simulink model "program_flight"  (R2017a)
settings: Solver=ode4  StartTime=0.0  StopTime=10  FixedStep=0.001  RelTol=1e-3
InitFcn:
  | BeforeSim
values from neighbouring files (symbols this model uses):
  S_ref = pi*(0.5*d_ref)^2    (= 0.0702153812059)    [BeforeSim.m]
libraries: simulink_need_slupdate x12, simulink x1
settings Model: Creator=Hans  LastModifiedBy=hhz
settings OptimizationCC: LifeSpan=inf
settings DebuggingCC: SFExecutionAtInitializationDiag=none
settings HardwareCC: ProdBitPerSizeT=32  ProdBitPerPtrDiffT=32  ProdWordSize=32  ProdHWDeviceType=Specified

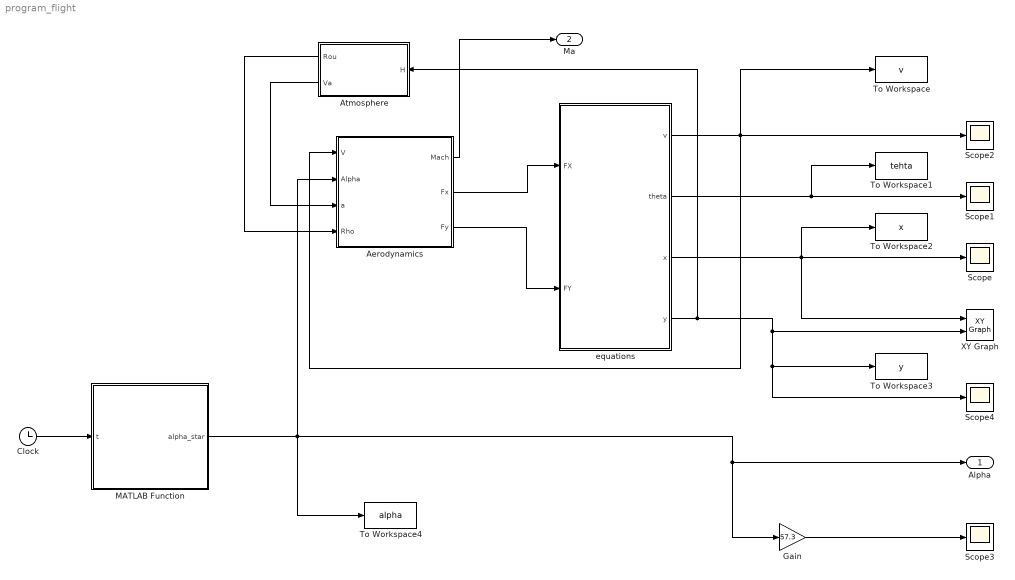
== system program_flight ==
  Aerodynamics : Subsystem
  Atmosphere : Subsystem
  Clock : Clock
  Gain : Gain  Gain=57.3
  MATLAB Function : MATLAB Function  TreatAsAtomicUnit=on
  Scope{,1..4} (5 alike) : Scope
  To Workspace : ToWorkspace  VariableName=v  SaveFormat=Timeseries  SampleTime=-1
  To Workspace1 : ToWorkspace  VariableName=tehta  SaveFormat=Timeseries  SampleTime=-1
  To Workspace2 : ToWorkspace  VariableName=x  SaveFormat=Timeseries  SampleTime=-1
  To Workspace3 : ToWorkspace  VariableName=y  SaveFormat=Timeseries  SampleTime=-1
  To Workspace4 : ToWorkspace  VariableName=alpha  SaveFormat=Timeseries  SampleTime=-1
  XY Graph : simulink/Sinks/XY Graph  xmin=0  xmax=3000  ymin=3000  ymax=4500  st=-1
  equations : Subsystem
  Alpha : Outport
  Ma : Outport  Port=2
  wires:
  Gain/1 -> Scope3/1
  equations/4(y) -> To Workspace3/1, Scope4/1, XY Graph/2, Atmosphere/1(H)
  equations/1(v) -> To Workspace/1, Scope2/1, Aerodynamics/1(V)
  Aerodynamics/1(" Mach") -> Ma/1
  Aerodynamics/2(Fx) -> equations/1(FX)
  Atmosphere/1(Rou) -> Aerodynamics/4(Rho)
  Aerodynamics/3(Fy) -> equations/2(FY)
  Atmosphere/2(Va) -> Aerodynamics/3(a)
  Clock/1 -> MATLAB Function/1(t)
  equations/2(theta) -> To Workspace1/1, Scope1/1
  equations/3(x) -> To Workspace2/1, XY Graph/1, Scope/1
  MATLAB Function/1(alpha_star) -> To Workspace4/1, Aerodynamics/2(Alpha), Alpha/1, Gain/1

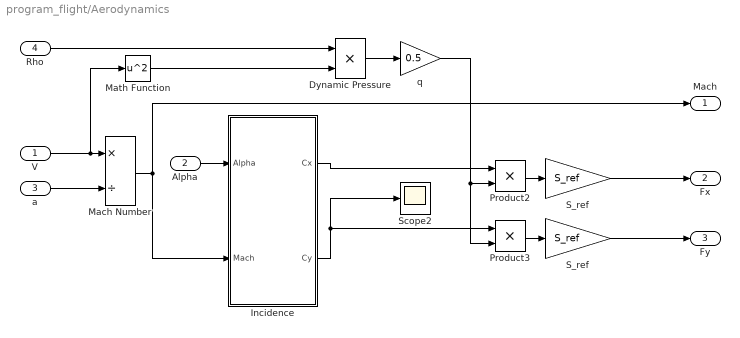
== system program_flight/Aerodynamics ==
  V : Inport
  Alpha : Inport  Port=2
  a : Inport  Port=3
  Rho : Inport  Port=4
  Dynamic Pressure : Product  SaturateOnIntegerOverflow=on  InputSameDT=on  OutDataTypeStr=Inherit: Same as first input
  Incidence : Subsystem
  Mach Number : Product  Inputs=*/  SaturateOnIntegerOverflow=on  InputSameDT=on  OutDataTypeStr=Inherit: Same as first input
  Math Function : Math  Operator=square  SaturateOnIntegerOverflow=on
  Product2 : Product  SaturateOnIntegerOverflow=on  InputSameDT=on  OutDataTypeStr=Inherit: Same as first input
  Product3 : Product  SaturateOnIntegerOverflow=on  InputSameDT=on  OutDataTypeStr=Inherit: Same as first input
  S_ref : Gain  Gain=S_ref  SaturateOnIntegerOverflow=on  OutDataTypeStr=Inherit: Same as input  ParamDataTypeStr=Inherit: Same as input
  "S_ref " : Gain  Gain=S_ref  SaturateOnIntegerOverflow=on  OutDataTypeStr=Inherit: Same as input  ParamDataTypeStr=Inherit: Same as input
  Scope2 : Scope
  q : Gain  Gain=0.5  SaturateOnIntegerOverflow=on  OutDataTypeStr=Inherit: Same as input  ParamDataTypeStr=Inherit: Same as input
  " Mach" : Outport  InitialOutput=0
  Fx : Outport  Port=2  InitialOutput=[0]
  Fy : Outport  Port=3  InitialOutput=0
  wires:
  Incidence/2(Cy) -> Product3/1, Scope2/1
  Product3/1 -> "S_ref "/1
  S_ref/1 -> Fx/1
  "S_ref "/1 -> Fy/1
  V/1 -> Math Function/1, Mach Number/1
  Alpha/1 -> Incidence/1(Alpha)
  Product2/1 -> S_ref/1
  Mach Number/1 -> " Mach"/1, Incidence/2(Mach)
  a/1 -> Mach Number/2
  q/1 -> Product2/2, Product3/2
  Rho/1 -> Dynamic Pressure/1
  Dynamic Pressure/1 -> q/1
  Math Function/1 -> Dynamic Pressure/2
  Incidence/1(Cx) -> Product2/1

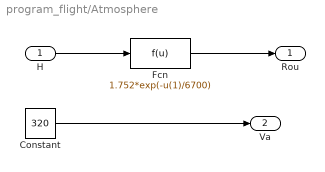
== system program_flight/Atmosphere ==
  H : Inport
  Constant : Constant  Value=320
  Fcn : Fcn  Expr=1.752*exp(-u(1)/6700)
  Rou : Outport
  Va : Outport  Port=2
  wires:
  H/1 -> Fcn/1
  Fcn/1 -> Rou/1
  Constant/1 -> Va/1

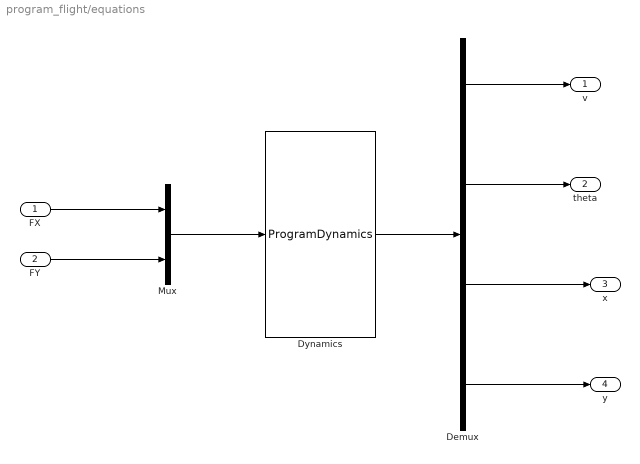
== system program_flight/equations ==
  FX : Inport
  FY : Inport  Port=2
  Demux : Demux
  Dynamics : S-Function  FunctionName=ProgramDynamics  SFunctionDeploymentMode=off  EnableBusSupport=off
  Mux : Mux  Inputs=2
  v : Outport
  theta : Outport  Port=2
  x : Outport  Port=3
  y : Outport  Port=4
  wires:
  FX/1 -> Mux/1
  FY/1 -> Mux/2
  Mux/1 -> Dynamics/1
  Dynamics/1 -> Demux/1
  Demux/1 -> v/1
  Demux/2 -> theta/1
  Demux/3 -> x/1
  Demux/4 -> y/1

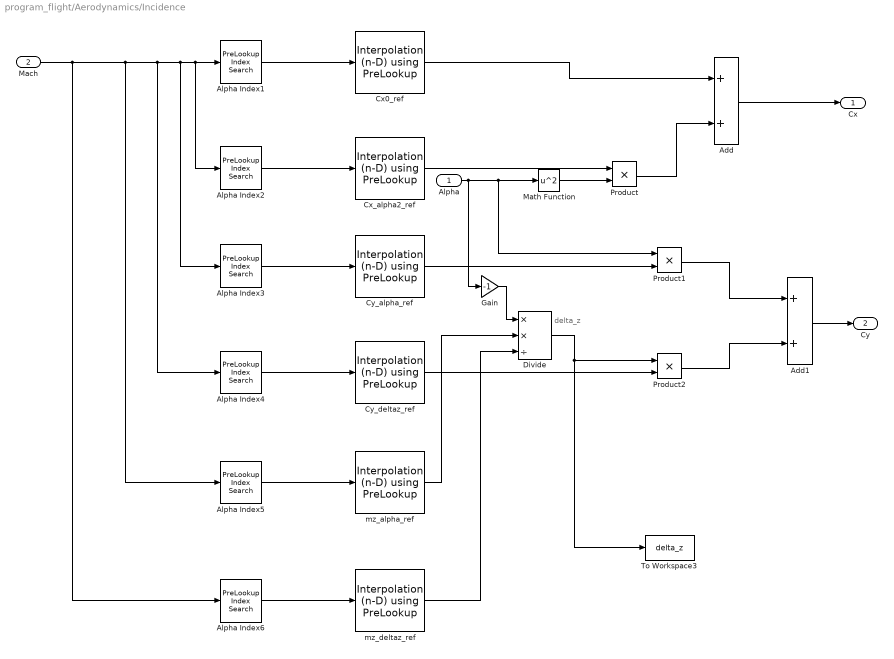
== system program_flight/Aerodynamics/Incidence ==
  note: delta_z
  Alpha : Inport
  Mach : Inport  Port=2
  Add : Sum
  Add1 : Sum
  Alpha Index{1..6} (6 alike) : simulink_need_slupdate/PreLookup Index Search  bpData=Mach_ref  searchMode=Binary Search  cacheBpFlag=on  outputFlag=off  IndexDataType=uint32  extrapMode=Linear Extrapolation  rangeErrorMode=None
      settings: SourceProductName=Simulink  SourceProductBaseCode=SL
  Cx0_ref : simulink_need_slupdate/Interpolation (n-D) using PreLookup  numDimsPopupSelect=1  explicitNumDims=2  table=Cx0_ref  interpMethod=Linear  extrapMethod=Linear  rangeErrorMode=None  NumSelectionDims=0
      settings: SourceProductName=Simulink  SourceProductBaseCode=SL
  Cx_alpha2_ref : simulink_need_slupdate/Interpolation (n-D) using PreLookup  numDimsPopupSelect=1  explicitNumDims=2  table=Cx_alpha2_ref  interpMethod=Linear  extrapMethod=Linear  rangeErrorMode=None  NumSelectionDims=0
      settings: SourceProductName=Simulink  SourceProductBaseCode=SL
  Cy_alpha_ref : simulink_need_slupdate/Interpolation (n-D) using PreLookup  numDimsPopupSelect=1  explicitNumDims=2  table=Cy_alpha_ref  interpMethod=Linear  extrapMethod=Linear  rangeErrorMode=None  NumSelectionDims=0
      settings: SourceProductName=Simulink  SourceProductBaseCode=SL
  Cy_deltaz_ref : simulink_need_slupdate/Interpolation (n-D) using PreLookup  numDimsPopupSelect=1  explicitNumDims=2  table=Cy_deltaz_ref  interpMethod=Linear  extrapMethod=Linear  rangeErrorMode=None  NumSelectionDims=0
      settings: SourceProductName=Simulink  SourceProductBaseCode=SL
  Divide : Product  Inputs=**/
  Gain : Gain  Gain=-1
  Math Function : Math  Operator=square  SaturateOnIntegerOverflow=on
  Product : Product
  Product1 : Product
  Product2 : Product
  To Workspace3 : ToWorkspace  VariableName=delta_z  SaveFormat=Timeseries  SampleTime=-1
  mz_alpha_ref : simulink_need_slupdate/Interpolation (n-D) using PreLookup  numDimsPopupSelect=1  explicitNumDims=2  table=mz_alpha_ref  interpMethod=Linear  extrapMethod=Linear  rangeErrorMode=None  NumSelectionDims=0
      settings: SourceProductName=Simulink  SourceProductBaseCode=SL
  mz_deltaz_ref : simulink_need_slupdate/Interpolation (n-D) using PreLookup  numDimsPopupSelect=1  explicitNumDims=2  table=mz_deltaz_ref  interpMethod=Linear  extrapMethod=Linear  rangeErrorMode=None  NumSelectionDims=0
      settings: SourceProductName=Simulink  SourceProductBaseCode=SL
  Cx : Outport  InitialOutput=0
  Cy : Outport  Port=2  InitialOutput=0
  wires:
  Alpha Index1/1 -> Cx0_ref/1
  Alpha Index2/1 -> Cx_alpha2_ref/1
  Alpha Index3/1 -> Cy_alpha_ref/1
  Alpha Index4/1 -> Cy_deltaz_ref/1
  Alpha Index5/1 -> mz_alpha_ref/1
  Alpha Index6/1 -> mz_deltaz_ref/1
  Mach/1 -> Alpha Index6/1, Alpha Index5/1, Alpha Index4/1, Alpha Index3/1, Alpha Index2/1, Alpha Index1/1
  Cx_alpha2_ref/1 -> Product/1
  Alpha/1 -> Gain/1, Product1/1, Math Function/1
  Math Function/1 -> Product/2
  Cx0_ref/1 -> Add/1
  Product/1 -> Add/2
  Add/1 -> Cx/1
  Cy_alpha_ref/1 -> Product1/2
  Divide/1 -> To Workspace3/1, Product2/1
  Cy_deltaz_ref/1 -> Product2/2
  Product1/1 -> Add1/1
  Product2/1 -> Add1/2
  Add1/1 -> Cy/1
  mz_alpha_ref/1 -> Divide/2
  mz_deltaz_ref/1 -> Divide/3
  Gain/1 -> Divide/1

== matlab function program_flight/MATLAB Function ==
  data: t input; alpha_star output
function alpha_star = fcn(t)
alpha_star_tem = 0;
if t > 0 && t < 3
    alpha_star_tem = 0;
else
    alpha_star_tem = 5;
end
alpha_star = alpha_star_tem*pi/180;%将度转换为弧度
